simulink model "battery_monitor"  (R2022b)
settings: Solver=FixedStepAuto  StartTime=0.0  StopTime=10.0  FixedStep=1e-3  RelTol=1e-3
libraries: battery_monitor_lib x1
settings Model: Creator=dr_pa  LastModifiedBy=dr_pa
settings DataIOCC: ExternalInput=BM1.getElement('GOV_e_bmCmd'),BM1.getElement('BM_b_prechrgContactorSts'),BM1.getElement('BM_b_HVposContactorSts'),BM1.getElement('BM_b_HVnegContactorSts')  LoadExternalInput=on

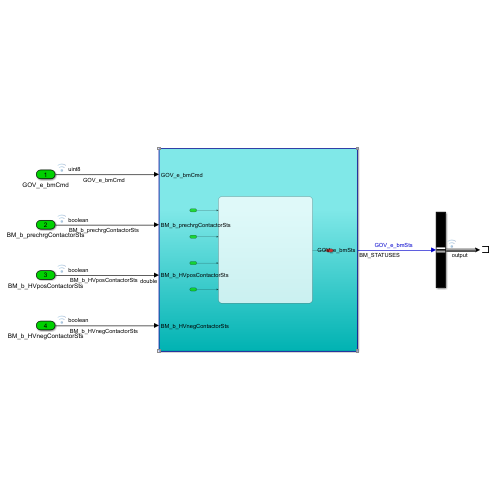
[thumbnail: Simulink's stored preview of the top-level diagram]
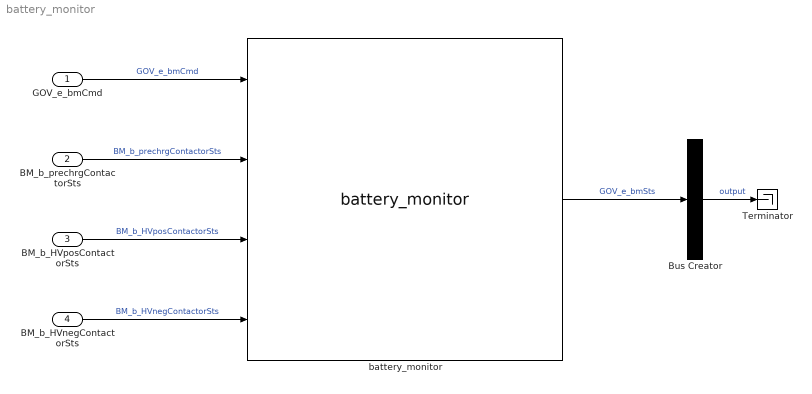
== system battery_monitor ==
  GOV_e_bmCmd : Inport  OutDataTypeStr=uint8  Interpolate=off
  BM_b_prechrgContactorSts : Inport  Port=2  OutDataTypeStr=boolean
  BM_b_HVposContactorSts : Inport  Port=3  OutDataTypeStr=boolean
  BM_b_HVnegContactorSts : Inport  Port=4  OutDataTypeStr=boolean
  Bus Creator : BusCreator  Inputs=1
  Terminator : Terminator
  battery_monitor : battery_monitor_lib/battery_monitor  SystemSampleTime=-1  VariantActivationTime=update diagram  Latency=0  AutoFrameSizeCalculation=off
  wires:
  battery_monitor/1 -> Bus Creator/1  "GOV_e_bmSts"
  Bus Creator/1 -> Terminator/1  "output"
  BM_b_HVposContactorSts/1 -> battery_monitor/3  "BM_b_HVposContactorSts"
  BM_b_HVnegContactorSts/1 -> battery_monitor/4  "BM_b_HVnegContactorSts"
  GOV_e_bmCmd/1 -> battery_monitor/1  "GOV_e_bmCmd"
  BM_b_prechrgContactorSts/1 -> battery_monitor/2  "BM_b_prechrgContactorSts"
